simulink model "simulinkm2"  (R2020b)
settings: Solver=VariableStepAuto  StartTime=0.0  StopTime=10.0  RelTol=1e-3
(part 1 of 5)
settings Model: Creator=shiel  LastModifiedBy=shiel

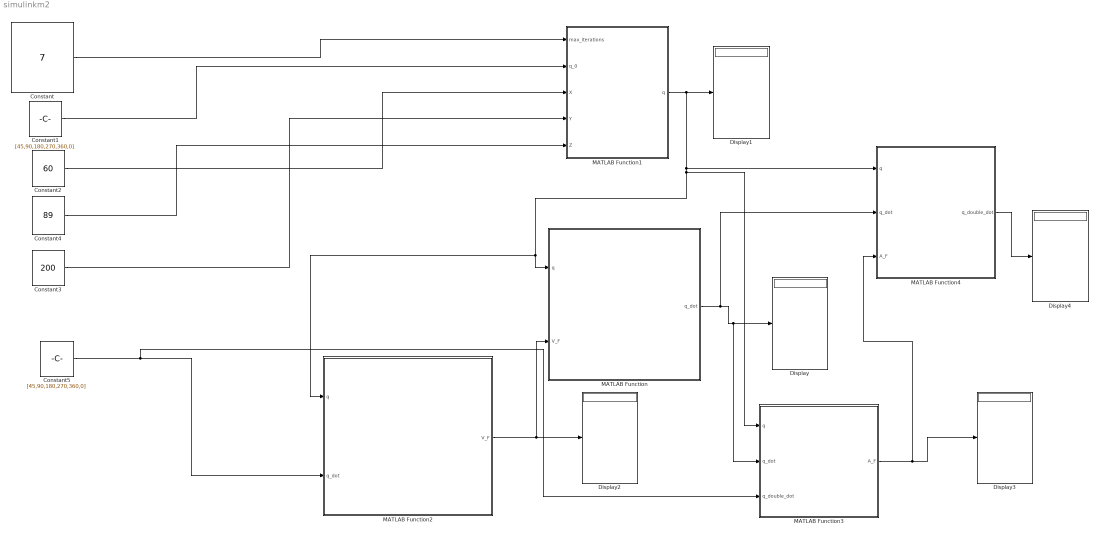
== system simulinkm2 ==
  Constant : Constant  Value=7
  Constant1 : Constant  Value=[45,90,180,270,360,0]
  Constant2 : Constant  Value=60
  Constant3 : Constant  Value=200
  Constant4 : Constant  Value=89
  Constant5 : Constant  Value=[45,90,180,270,360,0]
  Display{,1..4} (5 alike) : Display
  MATLAB Function : MATLAB Function  TreatAsAtomicUnit=on
  MATLAB Function1 : MATLAB Function  TreatAsAtomicUnit=on
  MATLAB Function2 : MATLAB Function  TreatAsAtomicUnit=on
  MATLAB Function3 : MATLAB Function  TreatAsAtomicUnit=on
  MATLAB Function4 : MATLAB Function  TreatAsAtomicUnit=on
  wires:
  MATLAB Function/1(q_dot) -> MATLAB Function4/2(q_dot), MATLAB Function3/2(q_dot), Display/1
  Constant/1 -> MATLAB Function1/1(max_iterations)
  Constant1/1 -> MATLAB Function1/2(q_0)
  Constant2/1 -> MATLAB Function1/3(X)
  Constant3/1 -> MATLAB Function1/4(Y)
  Constant4/1 -> MATLAB Function1/5(Z)
  MATLAB Function1/1(q) -> MATLAB Function4/1(q), MATLAB Function3/1(q), MATLAB Function2/1(q), MATLAB Function/1(q), Display1/1
  MATLAB Function2/1(V_F) -> MATLAB Function/2(V_F), Display2/1
  Constant5/1 -> MATLAB Function3/3(q_double_dot), MATLAB Function2/2(q_dot)
  MATLAB Function3/1(A_F) -> MATLAB Function4/3(A_F), Display3/1
  MATLAB Function4/1(q_double_dot) -> Display4/1

== matlab function simulinkm2/MATLAB Function1 ==
  data: max_iterations input; q output; q_0 input; X input; Y input; Z input
function q = inverse_position_kinematics(max_iterations, q_0, X,Y,Z)
  
      q_0=[q_0(1);q_0(2); q_0(3); q_0(4);q_0(5);q_0(6)];
     P = [X ; Y; Z]
      q_i=[q_0(1);q_0(2); q_0(3); q_0(4);q_0(5);q_0(6)];
      q1 = q_i(1);
      q2 = q_i(2);
      q3 = q_i(3);
      q4 = q_i(4);
      q5 = q_i(5);
      q6 = q_i(6);
      
      
       H=[10*sin((pi*q5)/180)*((pi*cos((pi*q1)/180)*sin((pi*q4)/180))/180 - (pi*cos((pi*q2)/180)*cos((pi*q3)/180)*cos((pi*q4)/180)*sin((pi*q1)/180))/180 + (pi*cos((pi*q4)/180)*sin((pi*q1)/180)*sin((pi*q2)/180)*sin((pi*q3)/180))/180) - (pi*sin((pi*q1)/180))/36 - (pi*cos((pi*q2)/180)*sin((pi*q1)/180))/36 - (pi*sin((pi*(q2 + q3))/180)*cos((pi*q5)/180)*sin((pi*q1)/180))/18 - (pi*cos((pi*q2)/180)*sin((pi*q1)/180)*sin((pi*q3)/180))/18 - (pi*cos((pi*q3)/180)*sin((pi*q1)/180)*sin((pi*q2)/180))/18, (pi*cos((pi*(q2 + q3))/180)*cos((pi*q1)/180)*cos((pi*q5)/180))/18 - (pi*cos((pi*q1)/180)*sin((pi*q2)/180))/36 - 10*sin((pi*q5)/180)*((pi*cos((pi*q1)/180)*cos((pi*q2)/180)*cos((pi*q4)/180)*sin((pi*q3)/180))/180 + (pi*cos((pi*q1)/180)*cos((pi*q3)/180)*cos((pi*q4)/180)*sin((pi*q2)/180))/180) + (pi*cos((pi*q1)/180)*cos((pi*q2)/180)*cos((pi*q3)/180))/18 - (pi*cos((pi*q1)/180)*sin((pi*q2)/180)*sin((pi*q3)/180))/18, (pi*cos((pi*(q2 + q3))/180)*cos((pi*q1)/180)*cos((pi*q5)/180))/18 - 10*sin((pi*q5)/180)*((pi*cos((pi*q1)/180)*cos((pi*q2)/180)*cos((pi*q4)/180)*sin((pi*q3)/180))/180 + (pi*cos((pi*q1)/180)*cos((pi*q3)/180)*cos((pi*q4)/180)*sin((pi*q2)/180))/180) + (pi*cos((pi*q1)/180)*cos((pi*q2)/180)*cos((pi*q3)/180))/18 - (pi*cos((pi*q1)/180)*sin((pi*q2)/180)*sin((pi*q3)/180))/18,  10*sin((pi*q5)/180)*((pi*cos((pi*q4)/180)*sin((pi*q1)/180))/180 - (pi*cos((pi*q1)/180)*cos((pi*q2)/180)*cos((pi*q3)/180)*sin((pi*q4)/180))/180 + (pi*cos((pi*q1)/180)*sin((pi*q2)/180)*sin((pi*q3)/180)*sin((pi*q4)/180))/180),   (pi*cos((pi*q5)/180)*(sin((pi*q1)/180)*sin((pi*q4)/180) + cos((pi*q1)/180)*cos((pi*q2)/180)*cos((pi*q3)/180)*cos((pi*q4)/180) - cos((pi*q1)/180)*cos((pi*q4)/180)*sin((pi*q2)/180)*sin((pi*q3)/180)))/18 - (pi*sin((pi*(q2 + q3))/180)*cos((pi*q1)/180)*sin((pi*q5)/180))/18, 0
(pi*cos((pi*q1)/180))/36 + 10*sin((pi*q5)/180)*((pi*sin((pi*q1)/180)*sin((pi*q4)/180))/180 + (pi*cos((pi*q1)/180)*cos((pi*q2)/180)*cos((pi*q3)/180)*cos((pi*q4)/180))/180 - (pi*cos((pi*q1)/180)*cos((pi*q4)/180)*sin((pi*q2)/180)*sin((pi*q3)/180))/180) + (pi*cos((pi*q1)/180)*cos((pi*q2)/180))/36 + (pi*sin((pi*(q2 + q3))/180)*cos((pi*q1)/180)*cos((pi*q5)/180))/18 + (pi*cos((pi*q1)/180)*cos((pi*q2)/180)*sin((pi*q3)/180))/18 + (pi*cos((pi*q1)/180)*cos((pi*q3)/180)*sin((pi*q2)/180))/18, (pi*cos((pi*(q2 + q3))/180)*cos((pi*q5)/180)*sin((pi*q1)/180))/18 - (pi*sin((pi*q1)/180)*sin((pi*q2)/180))/36 - 10*sin((pi*q5)/180)*((pi*cos((pi*q2)/180)*cos((pi*q4)/180)*sin((pi*q1)/180)*sin((pi*q3)/180))/180 + (pi*cos((pi*q3)/180)*cos((pi*q4)/180)*sin((pi*q1)/180)*sin((pi*q2)/180))/180) + (pi*cos((pi*q2)/180)*cos((pi*q3)/180)*sin((pi*q1)/180))/18 - (pi*sin((pi*q1)/180)*sin((pi*q2)/180)*sin((pi*q3)/180))/18, (pi*cos((pi*(q2 + q3))/180)*cos((pi*q5)/180)*sin((pi*q1)/180))/18 - 10*sin((pi*q5)/180)*((pi*cos((pi*q2)/180)*cos((pi*q4)/180)*sin((pi*q1)/180)*sin((pi*q3)/180))/180 + (pi*cos((pi*q3)/180)*cos((pi*q4)/180)*sin((pi*q1)/180)*sin((pi*q2)/180))/180) + (pi*cos((pi*q2)/180)*cos((pi*q3)/180)*sin((pi*q1)/180))/18 - (pi*sin((pi*q1)/180)*sin((pi*q2)/180)*sin((pi*q3)/180))/18, -10*sin((pi*q5)/180)*((pi*cos((pi*q1)/180)*cos((pi*q4)/180))/180 - (pi*sin((pi*q1)/180)*sin((pi*q2)/180)*sin((pi*q3)/180)*sin((pi*q4)/180))/180 + (pi*cos((pi*q2)/180)*cos((pi*q3)/180)*sin((pi*q1)/180)*sin((pi*q4)/180))/180), - (pi*cos((pi*q5)/180)*(cos((pi*q1)/180)*sin((pi*q4)/180) - cos((pi*q2)/180)*cos((pi*q3)/180)*cos((pi*q4)/180)*sin((pi*q1)/180) + cos((pi*q4)/180)*sin((pi*q1)/180)*sin((pi*q2)/180)*sin((pi*q3)/180)))/18 - (pi*sin((pi*(q2 + q3))/180)*sin((pi*q1)/180)*sin((pi*q5)/180))/18, 0
                                                                                                                                                                                                                                                                                                                                                                                                                                                                                                  0,                                                                                                                                                                                           (pi*sin((pi*(q2 + q3))/180))/18 + (pi*cos((pi*q2)/180))/36 + (pi*cos((pi*(q2 + q3))/180)*sin((pi*(q4 + q5))/180))/36 + (pi*sin((pi*(q2 + q3))/180)*cos((pi*q5)/180))/18 - (pi*cos((pi*(q2 + q3))/180)*sin((pi*(q4 - q5))/180))/36,                                                                                                                                                                          (pi*sin((pi*(q2 + q3))/180))/18 + (pi*cos((pi*(q2 + q3))/180)*sin((pi*(q4 + q5))/180))/36 + (pi*sin((pi*(q2 + q3))/180)*cos((pi*q5)/180))/18 - (pi*cos((pi*(q2 + q3))/180)*sin((pi*(q4 - q5))/180))/36,                                                                                                               (pi*cos((pi*(q4 + q5))/180)*sin((pi*(q2 + q3))/180))/36 - (pi*sin((pi*(q2 + q3))/180)*cos((pi*(q4 - q5))/180))/36,                                                                                                           (pi*cos((pi*(q4 + q5))/180)*sin((pi*(q2 + q3))/180))/36 + (pi*cos((pi*(q2 + q3))/180)*sin((pi*q5)/180))/18 + (pi*sin((pi*(q2 + q3))/180)*cos((pi*(q4 - q5))/180))/36, 0];
                                                                                                                                                                                                                                                                                                                                                                                                                                                                                              
                                                                                                                                                                                                                                                                                                                                                                                                                                                                                              
    
     
     
   
    q2= pinv(H)*P;
     q_i = q_i - q2 ;
      
      
   for   i = 0 : max_iterations 
     
  
   
  
     q1 = q_i(1);
      q2 = q_i(2);
      q3 = q_i(3);
      q4 = q_i(4);
      q5 = q_i(5);
      q6 = q_i(6);
      
      
       H=[10*sin((pi*q5)/180)*((pi*cos((pi*q1)/180)*sin((pi*q4)/180))/180 - (pi*cos((pi*q2)/180)*cos((pi*q3)/180)*cos((pi*q4)/180)*sin((pi*q1)/180))/180 + (pi*cos((pi*q4)/180)*sin((pi*q1)/180)*sin((pi*q2)/180)*sin((pi*q3)/180))/180) - (pi*sin((pi*q1)/180))/36 - (pi*cos((pi*q2)/180)*sin((pi*q1)/180))/36 - (pi*sin((pi*(q2 + q3))/180)*cos((pi*q5)/180)*sin((pi*q1)/180))/18 - (pi*cos((pi*q2)/180)*sin((pi*q1)/180)*sin((pi*q3)/180))/18 - (pi*cos((pi*q3)/180)*sin((pi*q1)/180)*sin((pi*q2)/180))/18, (pi*cos((pi*(q2 + q3))/180)*cos((pi*q1)/180)*cos((pi*q5)/180))/18 - (pi*cos((pi*q1)/180)*sin((pi*q2)/180))/36 - 10*sin((pi*q5)/180)*((pi*cos((pi*q1)/180)*cos((pi*q2)/180)*cos((pi*q4)/180)*sin((pi*q3)/180))/180 + (pi*cos((pi*q1)/180)*cos((pi*q3)/180)*cos((pi*q4)/180)*sin((pi*q2)/180))/180) + (pi*cos((pi*q1)/180)*cos((pi*q2)/180)*cos((pi*q3)/180))/18 - (pi*cos((pi*q1)/180)*sin((pi*q2)/180)*sin((pi*q3)/180))/18, (pi*cos((pi*(q2 + q3))/180)*cos((pi*q1)/180)*cos((pi*q5)/180))/18 - 10*sin((pi*q5)/180)*((pi*cos((pi*q1)/180)*cos((pi*q2)/180)*cos((pi*q4)/180)*sin((pi*q3)/180))/180 + (pi*cos((pi*q1)/180)*cos((pi*q3)/180)*cos((pi*q4)/180)*sin((pi*q2)/180))/180) + (pi*cos((pi*q1)/180)*cos((pi*q2)/180)*cos((pi*q3)/180))/18 - (pi*cos((pi*q1)/180)*sin((pi*q2)/180)*sin((pi*q3)/180))/18,  10*sin((pi*q5)/180)*((pi*cos((pi*q4)/180)*sin((pi*q1)/180))/180 - (pi*cos((pi*q1)/180)*cos((pi*q2)/180)*cos((pi*q3)/180)*sin((pi*q4)/180))/180 + (pi*cos((pi*q1)/180)*sin((pi*q2)/180)*sin((pi*q3)/180)*sin((pi*q4)/180))/180),   (pi*cos((pi*q5)/180)*(sin((pi*q1)/180)*sin((pi*q4)/180) + cos((pi*q1)/180)*cos((pi*q2)/180)*cos((pi*q3)/180)*cos((pi*q4)/180) - cos((pi*q1)/180)*cos((pi*q4)/180)*sin((pi*q2)/180)*sin((pi*q3)/180)))/18 - (pi*sin((pi*(q2 + q3))/180)*cos((pi*q1)/180)*sin((pi*q5)/180))/18, 0
(pi*cos((pi*q1)/180))/36 + 10*sin((pi*q5)/180)*((pi*sin((pi*q1)/180)*sin((pi*q4)/180))/180 + (pi*cos((pi*q1)/180)*cos((pi*q2)/180)*cos((pi*q3)/180)*cos((pi*q4)/180))/180 - (pi*cos((pi*q1)/180)*cos((pi*q4)/180)*sin((pi*q2)/180)*sin((pi*q3)/180))/180) + (pi*cos((pi*q1)/180)*cos((pi*q2)/180))/36 + (pi*sin((pi*(q2 + q3))/180)*cos((pi*q1)/180)*cos((pi*q5)/180))/18 + (pi*cos((pi*q1)/180)*cos((pi*q2)/180)*sin((pi*q3)/180))/18 + (pi*cos((pi*q1)/180)*cos((pi*q3)/180)*sin((pi*q2)/180))/18, (pi*cos((pi*(q2 + q3))/180)*cos((pi*q5)/180)*sin((pi*q1)/180))/18 - (pi*sin((pi*q1)/180)*sin((pi*q2)/180))/36 - 10*sin((pi*q5)/180)*((pi*cos((pi*q2)/180)*cos((pi*q4)/180)*sin((pi*q1)/180)*sin((pi*q3)/180))/180 + (pi*cos((pi*q3)/180)*cos((pi*q4)/180)*sin((pi*q1)/180)*sin((pi*q2)/180))/180) + (pi*cos((pi*q2)/180)*cos((pi*q3)/180)*sin((pi*q1)/180))/18 - (pi*sin((pi*q1)/180)*sin((pi*q2)/180)*sin((pi*q3)/180))/18, (pi*cos((pi*(q2 + q3))/180)*cos((pi*q5)/180)*sin((pi*q1)/180))/18 - 10*sin((pi*q5)/180)*((pi*cos((pi*q2)/180)*cos((pi*q4)/180)*sin((pi*q1)/180)*sin((pi*q3)/180))/180 + (pi*cos((pi*q3)/180)*cos((pi*q4)/180)*sin((pi*q1)/180)*sin((pi*q2)/180))/180) + (pi*cos((pi*q2)/180)*cos((pi*q3)/180)*sin((pi*q1)/180))/18 - (pi*sin((pi*q1)/180)*sin((pi*q2)/180)*sin((pi*q3)/180))/18, -10*sin((pi*q5)/180)*((pi*cos((pi*q1)/180)*cos((pi*q4)/180))/180 - (pi*sin((pi*q1)/180)*sin((pi*q2)/180)*sin((pi*q3)/180)*sin((pi*q4)/180))/180 + (pi*cos((pi*q2)/180)*cos((pi*q3)/180)*sin((pi*q1)/180)*sin((pi*q4)/180))/180), - (pi*cos((pi*q5)/180)*(cos((pi*q1)/180)*sin((pi*q4)/180) - cos((pi*q2)/180)*cos((pi*q3)/180)*cos((pi*q4)/180)*sin((pi*q1)/180) + cos((pi*q4)/180)*sin((pi*q1)/180)*sin((pi*q2)/180)*sin((pi*q3)/180)))/18 - (pi*sin((pi*(q2 + q3))/180)*sin((pi*q1)/180)*sin((pi*q5)/180))/18, 0
                                                                                                                                                                                                                                                                                                                                                                                                                                                                                                  0,                                                                                                                                                                                           (pi*sin((pi*(q2 + q3))/180))/18 + (pi*cos((pi*q2)/180))/36 + (pi*cos((pi*(q2 + q3))/180)*sin((pi*(q4 + q5))/180))/36 + (pi*sin((pi*(q2 + q3))/180)*cos((pi*q5)/180))/18 - (pi*cos((pi*(q2 + q3))/180)*sin((pi*(q4 - q5))/180))/36,                                                                                                                                                                          (pi*sin((pi*(q2 + q3))/180))/18 + (pi*cos((pi*(q2 + q3))/180)*sin((pi*(q4 + q5))/180))/36 + (pi*sin((pi*(q2 + q3))/180)*cos((pi*q5)/180))/18 - (pi*cos((pi*(q2 + q3))/180)*sin((pi*(q4 - q5))/180))/36,                                                                                                               (pi*cos((pi*(q4 + q5))/180)*sin((pi*(q2 + q3))/180))/36 - (pi*sin((pi*(q2 + q3))/180)*cos((pi*(q4 - q5))/180))/36,                                                                                                           (pi*cos((pi*(q4 + q5))/180)*sin((pi*(q2 + q3))/180))/36 + (pi*cos((pi*(q2 + q3))/180)*sin((pi*q5)/180))/18 + (pi*sin((pi*(q2 + q3))/180)*cos((pi*(q4 - q5))/180))/36, 0];
                                                                                                                                                                                                                                                                                                                                                                                                                                                                                              
                                                                                                                                                                                                                                                                                                                                                                                                                                                                                              
    
     
     
      
    q2= pinv(H)*P ;
     q_i = q_i - q2 ;
       
               
   end
   q = q_i
end
